simulink model "controller"  (R2021b)
settings: Solver=FixedStepDiscrete  StartTime=0.0  StopTime=10.0  FixedStep=0.001  RelTol=1e-3  EnableMultiTasking=on
libraries: simulink x4
settings Model: PacingRate=3  ExtModeTrigDuration=2  Creator=DAUIN-Win10  LastModifiedBy=gianlucalm
settings DataIOCC: SaveOutput=off  SaveTime=off
settings OptimizationCC: EnhancedBackFolding=on  PassReuseOutputArgsAs=Individual arguments  MaxStackSize=64  OptimizeBlockOrder=speed  DifferentSizesBufferReuse=on  OptimizationCustomize=off  EfficientTunableParamExpr=on
settings DebuggingCC: ParameterTunabilityLossMsg=error
settings HardwareCC: ProdBitPerInt=16  ProdBitPerPointer=16  ProdBitPerSizeT=16  ProdBitPerPtrDiffT=16  ProdLargestAtomicFloat=None  ProdWordSize=8  ProdHWDeviceType=Atmel->AVR
settings SFSimCC: MATLABDynamicMemAlloc=off
settings RTWCC: Description=Embedded Coder  SystemTargetFile=ert.tlc  HardwareBoard=Arduino Uno  GenCodeOnly=on  TemplateMakefile=ert_default_tmf  Toolchain=Arduino AVR  BuildConfiguration=Faster Runs
settings CodeAppCC: ForceParamTrailComments=on  IgnoreCustomStorageClasses=off  OperatorAnnotations=on  SimulinkDataObjDesc=on  SFDataObjDesc=on  InsertBlockDesc=on
settings ERTTargetCC: CodeInterfacePackaging=Reusable function  SupportContinuousTime=on  SupportVariableSizeSignals=on  ExtModeTransport=3  ExtModeStaticAlloc=on  ExtModeStaticAllocSize=250  ExtModeMexFile=ext_xcp  ExtModeIntrfLevel=Level2 - Open  ERTFilePackagingFormat=Compact

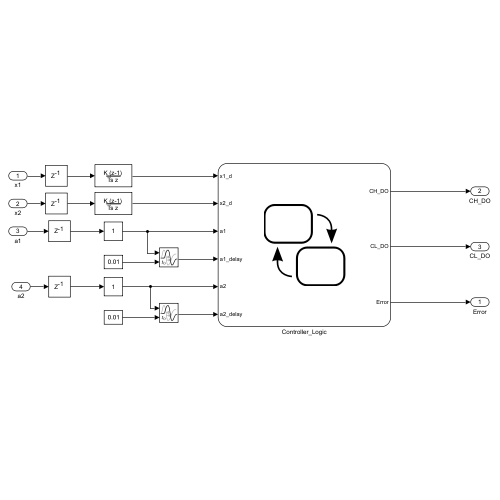
[thumbnail: Simulink's stored preview of the top-level diagram]
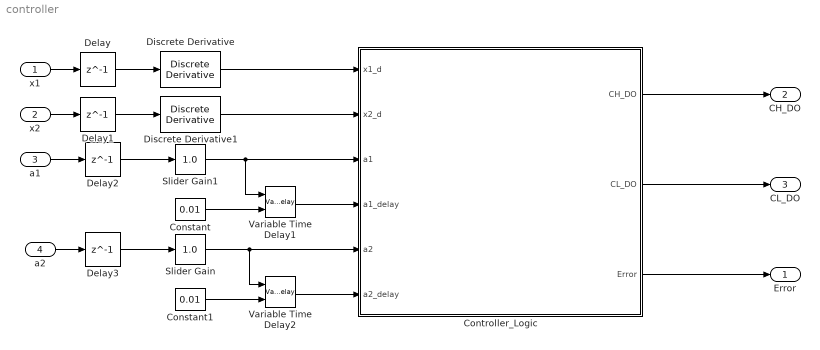
== system controller ==
  x1 : Inport
  x2 : Inport  Port=2
  a1 : Inport  Port=3
  a2 : Inport  Port=4
  Constant : Constant  Value=0.01
  Constant1 : Constant  Value=0.01
  Controller_Logic : Stateflow chart  TreatAsAtomicUnit=on
      settings: PortSchema="{\"entries\":[{\"content\":{\"sides\":[{\"content\":{\"connectorIds\":[\"In1\",\"In2\",\"In5\",\"In3\",\"In6\",\"In4\"]},\"type\":\"ConnectorPlacement.EquallySpacedRectSide\",\"uuid\":\"03fcdeea-861d-403d-a713-017c2a853cd0\"},{\"content\":{\"connectorIds\":[\"Out1\",\"Out2\",\"Out3\"],\"side\":\"RIGHT\"},\"type\":\"ConnectorPlacement.EquallySpacedRectSide\",\"uuid\":\"c533f712-70b6-4dd9-9569-6aad03cb8087\"},{\"content\":{\"connectorIds\":[],\"side\":\"TOP\"},\"type\":\"ConnectorPlacement.EquallySpacedRectSide\",\"uuid\":\"58c96a87-d27c-4904-8775-afc8acbd3a66\"}]},\"type\":\"ConnectorPlacement.EquallySpacedConnector\",\"uuid\":\"db3d0038-3e4d-416e-9575-e84c800f913b\"}],\"packageUris\":[\"http://schema.mathworks.com/mf0/Connector/R2020b\"],\"version\":\"1.0\"}"
  Delay{,1..3} (4 alike) : Delay  DelayLength=1  InitialCondition=0
  Discrete Derivative : simulink/Discrete/Discrete Derivative  gainval=1.0  ICPrevScaledInput=0.0  OutMin=[]  OutMax=[]  OutDataType=fixdt(1, 16)  OutScaling=2^-10  DoSatur=off
  Discrete Derivative1 : simulink/Discrete/Discrete Derivative  gainval=1.0  ICPrevScaledInput=0.0  OutMin=[]  OutMax=[]  OutDataType=fixdt(1, 16)  OutScaling=2^-10  DoSatur=off
  Slider Gain : simulink/Math Operations/Slider Gain  gain=1.0  low=0  high=1
  Slider Gain1 : simulink/Math Operations/Slider Gain  gain=1.0  low=0  high=1
  Variable Time Delay1 : VariableTransportDelay  MaximumDelay=10  MaximumPoints=10240
  Variable Time Delay2 : VariableTransportDelay  MaximumDelay=10  MaximumPoints=10240
  Error : Outport  OutDataTypeStr=boolean
  CH_DO : Outport  Port=2  OutDataTypeStr=boolean
  CL_DO : Outport  Port=3  OutDataTypeStr=boolean
  wires:
  x2/1 -> Delay1/1
  x1/1 -> Delay/1
  Controller_Logic/1(CH_DO) -> CH_DO/1
  Controller_Logic/2(CL_DO) -> CL_DO/1
  Controller_Logic/3(Error) -> Error/1
  Delay/1 -> Discrete Derivative/1
  Delay1/1 -> Discrete Derivative1/1
  Variable Time Delay1/1 -> Controller_Logic/3(a1_delay)
  Variable Time Delay2/1 -> Controller_Logic/4(a2_delay)
  a1/1 -> Delay2/1
  Delay2/1 -> Slider Gain1/1
  Constant/1 -> Variable Time Delay1/2
  a2/1 -> Delay3/1
  Constant1/1 -> Variable Time Delay2/2
  Discrete Derivative/1 -> Controller_Logic/1(x1_d)
  Discrete Derivative1/1 -> Controller_Logic/2(x2_d)
  Slider Gain1/1 -> Controller_Logic/5(a1), Variable Time Delay1/1
  Delay3/1 -> Slider Gain/1
  Slider Gain/1 -> Variable Time Delay2/1, Controller_Logic/6(a2)

== stateflow chart controller/Controller_Logic ==
  state On_Off_Logic [parallel]
    settings: executionOrder=1
    state OFF
      en:
      CH_DO = 1;
      CL_DO = 0;
    state ON
      during: XTable(x1_d,x2_d)
    (default) -> OFF
    OFF -> ON : [Safe_State==0]
    ON -> OFF : [Safe_State==1]
  state Error_Logic [parallel]
    settings: executionOrder=2
    state OK
      en:
      Error = 0;
      Safe_State= 0;
    state ERROR
      en:
      Error = 1;
      Safe_State=1;
    (default) -> OK
    OK -> ERROR : [duration(NotChange(a1, a1_delay),msec)>=20 || duration(NotChange(a2, a2_delay),msec)>=20]
  data: v1 function_input double; v2 function_input double; a_now function_input double; a_after function_input double; f function_output double; CH_DO output boolean; CL_DO output boolean; x1_d input double; x2_d input double; Error output boolean; Safe_State local double; a1_delay input double size=1; a2_delay input double size=1; a1 input double size=1; a2 input double size=1
  function XTable(v1,v2):
    | function XTable(v1,v2)
    | 
    | aVarTruthTableCondition_1 = false;
    | aVarTruthTableCondition_2 = false;
    | 
    | 
    | % More comfort is given to the driver by switching the softer damping factor.
    | 
    | aVarTruthTableCondition_1 = logical((v1 - v2) * v1< 0);
    | 
    | % More reactivity is given to the driver by switching the harder damping factor.
    | 
    | aVarTruthTableCondition_2 = logical((v1 - v2) * v1 >= 0);
    | 
    | if (aVarTruthTableCondition_1 && ~aVarTruthTableCondition_2)
    |     A2();
    | elseif (~aVarTruthTableCondition_1 && aVarTruthTableCondition_2)
    |     A1();
    | else % Default
    |     A1();
    | end
    | 
    | function A1()
    | 
    | % Switch to harder damping factor
    | 
    | CH_DO = true;CL_DO = false;
    | 
    | function A2()
    | 
    | % Switch to softer damping factor
    | 
    | CH_DO = false;CL_DO = true;
  function f=NotChange(a_now, a_after):
    | function f=NotChange(a_now, a_after)
    |     if abs(a_now-a_after)< 1e-5 
    |         f=1;
    |     else
    |         f=0;
    |     end
    | end
